simulink model "OU"  (R2021b)
settings: Solver=VariableStepAuto  StartTime=0.0  StopTime=15  RelTol=1e-3
undefined symbols (not defined in the file or in its folder): denum, num
settings Model: Creator=vkad  LastModifiedBy=vkad

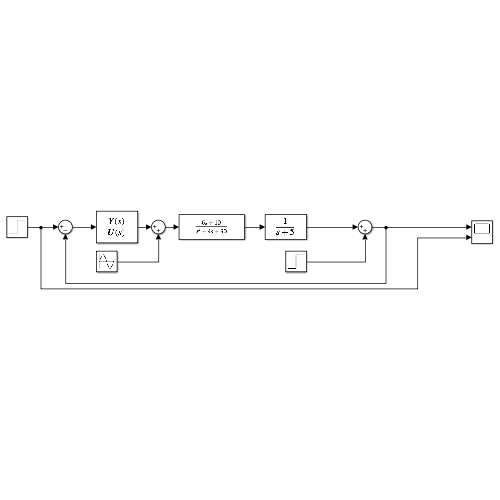
[thumbnail: Simulink's stored preview of the top-level diagram]
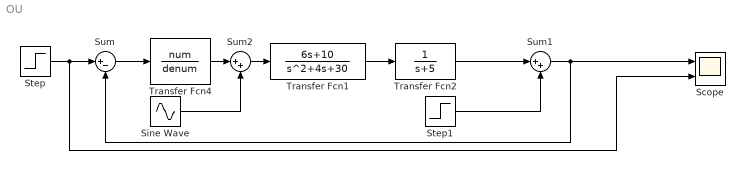
== system OU ==
  Scope : Scope  NumInputPorts=2
  Sine Wave : Sin  Amplitude=0.1  Frequency=0.5  SampleTime=0
  Step : Step  Time=0  After=0.5  SampleTime=0
  Step1 : Step  Time=0  After=0.15  SampleTime=0
  Sum : Sum  Inputs=|+-
  Sum1 : Sum  Inputs=|++
  Sum2 : Sum  Inputs=|++
  Transfer Fcn1 : TransferFcn  Numerator=[6 10]  Denominator=[1 4 30]
  Transfer Fcn2 : TransferFcn  Denominator=[1 5]
  Transfer Fcn4 : TransferFcn  Numerator=num  Denominator=denum
  wires:
  Sum/1 -> Transfer Fcn4/1
  Step/1 -> Scope/2, Sum/1
  Transfer Fcn2/1 -> Sum1/1
  Sum1/1 -> Scope/1, Sum/2
  Transfer Fcn1/1 -> Transfer Fcn2/1
  Transfer Fcn4/1 -> Sum2/1
  Sum2/1 -> Transfer Fcn1/1
  Sine Wave/1 -> Sum2/2
  Step1/1 -> Sum1/2
